simulink model "suijibijin"  (Simulink 7.1)
settings: Solver=ode45  StartTime=0.0  StopTime=200  FixedStep=0.001  RelTol=1e-3  AbsTol=1e-3
libraries: simulink x9
settings Model: Creator=ThinkPad  LastModifiedBy=casi  ExtModeTrigMode=oneshot  ExtModeArmWhenConnect=off
settings DataIOCC: LimitDataPoints=off  SignalLoggingName=sigsOut
settings OptimizationCC: BooleanDataType=off
settings DebuggingCC: SaveWithParameterizedLinksMsg=none  SignalResolutionControl=TryResolveAllWithWarning  SolverPrmCheckMsg=none  MultiTaskDSMMsg=warning  MultiTaskCondExecSysMsg=none  StrictBusMsg=None
settings HardwareCC: TargetUnknown=on
settings RTWCC: IncludeERTFirstTime=on
settings GRTTargetCC: TargetFcnLib=ansi_tfl_tmw.mat

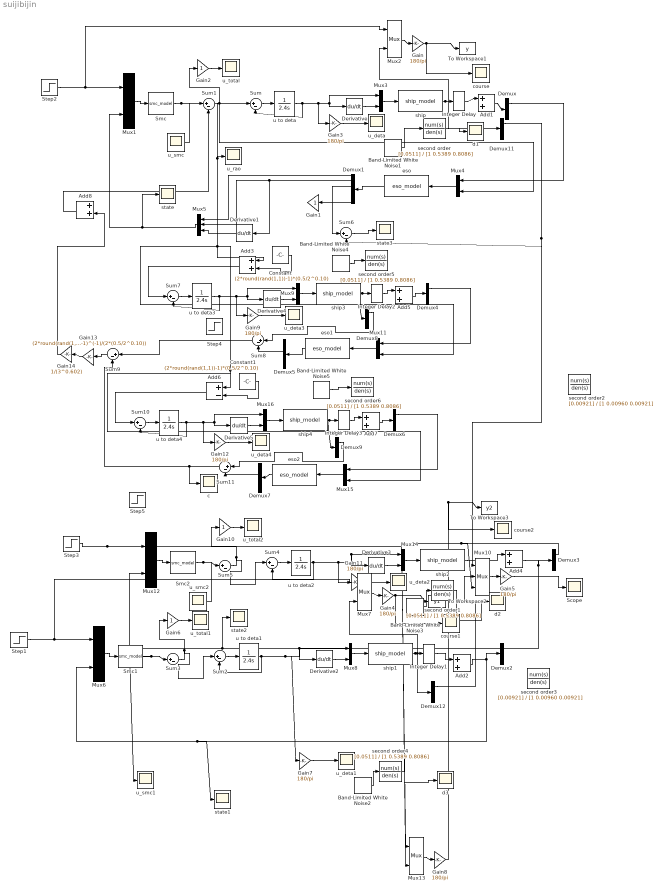
== system suijibijin ==
  Add{1..2,4..5,7} (5 alike) : Sum  OutDataType=sfix(16)  OutScaling=2^-10
  Add3 : Sum  Orientation=left  OutDataType=sfix(16)  OutScaling=2^-10
  Add6 : Sum  Orientation=left  Inputs=+-  OutDataType=sfix(16)  OutScaling=2^-10
  Add8 : Sum  Orientation=left  OutDataType=sfix(16)  OutScaling=2^-10
  Band-Limited White Noise{1..5} (5 alike) : simulink/Sources/Band-Limited White Noise  SystemSampleTime=-1  Cov=[0.01]  Ts=0.1  seed=[23341]
  Constant : Constant  Value=(2*round(rand(1,1))-1)*(0.5/2^0.10)  OutDataType=sfix(16)  OutScaling=2^0
  Constant1 : Constant  Value=(2*round(rand(1,1))-1)*(0.5/2^0.10)  OutDataType=sfix(16)  OutScaling=2^0
  Demux{,2..4,6,8..9,11..12} (9 alike) : Demux  Outputs=3
  Demux1 : Demux  Orientation=left  Outputs=6
  Demux5 : Demux  Orientation=left  Outputs=6
  Demux7 : Demux  Orientation=left  Outputs=6
  Derivative{,2..5} (5 alike) : Derivative
  Derivative1 : Derivative  Orientation=left
  Gain{,3..5,7..9,11..12} (9 alike) : Gain  Gain=180/pi  ParameterDataType=sfix(16)  ParameterScaling=2^0  OutDataType=sfix(16)  OutScaling=2^0
  Gain1 : Gain  Orientation=left  ParameterDataType=sfix(16)  ParameterScaling=2^0  OutDataType=sfix(16)  OutScaling=2^0
  Gain10 : Gain  ParameterDataType=sfix(16)  ParameterScaling=2^0  OutDataType=sfix(16)  OutScaling=2^0
  Gain13 : Gain  Orientation=left  Gain=(2*round(rand(1,1))-1)^(-1)/(2*(0.5/2^0.10))  ParameterDataType=sfix(16)  ParameterScaling=2^0  OutDataType=sfix(16)  OutScaling=2^0
  Gain14 : Gain  Orientation=left  Gain=1/(3^0.602)  ParameterDataType=sfix(16)  ParameterScaling=2^0  OutDataType=sfix(16)  OutScaling=2^0
  Gain2 : Gain  ParameterDataType=sfix(16)  ParameterScaling=2^0  OutDataType=sfix(16)  OutScaling=2^0
  Gain6 : Gain  ParameterDataType=sfix(16)  ParameterScaling=2^0  OutDataType=sfix(16)  OutScaling=2^0
  Integer Delay{,1..3} (4 alike) : simulink/Discrete/Integer Delay  vinit=0.0  samptime=-1  NumDelays=200
  Mux{1..3,6..9,12..14,16} (11 alike) : Mux  Inputs=2
  Mux10 : Mux  Inputs=3
  Mux11 : Mux  Orientation=left  Inputs=2
  Mux15 : Mux  Orientation=left  Inputs=2
  Mux4 : Mux  Orientation=left  Inputs=2
  Mux5 : Mux  Orientation=left  Inputs=3
  Scope : Scope
      settings: YMin=29.985  YMax=30.0125  SaveName=coursebijiao  DataFormat=Array
  Smc : S-Function  FunctionName=smc_model  EnableBusSupport=off
  Smc1 : S-Function  FunctionName=smc_model  EnableBusSupport=off
  Smc2 : S-Function  FunctionName=smc_model  EnableBusSupport=off
  Step1 : Step  Time=0  After=30*pi/180  SampleTime=0  ZeroCross=off
  Step2 : Step  Time=0  After=30*pi/180  SampleTime=0  ZeroCross=off
  Step3 : Step  Time=0  After=30*pi/180  SampleTime=0  ZeroCross=off
  Step4 : Step  Time=0  After=10*pi/180  SampleTime=0  ZeroCross=off
  Step5 : Step  Time=0  After=10*pi/180  SampleTime=0  ZeroCross=off
  Sum{,1..7,10} (9 alike) : Sum  Inputs=|+-  OutDataType=sfix(16)  OutScaling=2^0
  Sum11 : Sum  Orientation=left  Inputs=|+-  OutDataType=sfix(16)  OutScaling=2^0
  Sum8 : Sum  Orientation=left  Inputs=|+-  OutDataType=sfix(16)  OutScaling=2^0
  Sum9 : Sum  Orientation=left  Inputs=|+-  OutDataType=sfix(16)  OutScaling=2^0
  To Workspace1 : ToWorkspace  VariableName=y  SampleTime=-1  SaveFormat=Array
  To Workspace2 : ToWorkspace  VariableName=y1  SampleTime=-1  SaveFormat=Array
  To Workspace3 : ToWorkspace  VariableName=y2  SampleTime=-1  SaveFormat=Array
  c : Scope
      settings: YMin=-0.005  YMax=0.105  SaveName=course3  SampleInput=on
  course : Scope
      settings: YMin=-0.005  YMax=0.105  SaveName=course  SampleInput=on
  course1 : Scope
      settings: YMin=-0.005  YMax=0.105  SaveName=course1  SampleInput=on
  course2 : Scope
      settings: YMin=-0.005  YMax=0.105  SaveName=course2  SampleInput=on
  d1 : Scope
      settings: SaveName=u_total1  SampleInput=on
  d2 : Scope
      settings: SaveName=u_total4  SampleInput=on
  d3 : Scope
      settings: SaveName=u_total2  SampleInput=on
  eso : S-Function  Orientation=left  FunctionName=eso_model  EnableBusSupport=off
  eso1 : S-Function  Orientation=left  FunctionName=eso_model  EnableBusSupport=off
  eso2 : S-Function  Orientation=left  FunctionName=eso_model  EnableBusSupport=off
  second order{,1,4..6} (5 alike) : TransferFcn  Numerator=[0.0511]  Denominator=[1 0.5389 0.8086]
  second order2 : TransferFcn  Numerator=[0.00921]  Denominator=[1 0.00960 0.00921]
  second order3 : TransferFcn  Numerator=[0.00921]  Denominator=[1 0.00960 0.00921]
  ship{,1..4} (5 alike) : S-Function  FunctionName=ship_model  EnableBusSupport=off
  state{,1..3} (4 alike) : Scope
      state settings: SaveName=u_rao1  SampleInput=on
      state1 settings: SaveName=u_rao2  SampleInput=on
      state2 settings: SaveName=u_rao3  SampleInput=on
      state3 settings: SaveName=u_rao4  SampleInput=on
  u to deta{,1..4} (5 alike) : TransferFcn  Denominator=[2.4 0]
  u_deta{,1..4} (5 alike) : Scope
      u_deta settings: TimeRange=100  YMin=2.275e+014  YMax=2.365e+014  SaveName=u_deta  SampleInput=on
      u_deta1 settings: TimeRange=100  YMin=2.275e+014  YMax=2.365e+014  SaveName=u_deta1  SampleInput=on
      u_deta2 settings: TimeRange=100  YMin=2.275e+014  YMax=2.365e+014  SaveName=u_deta2  SampleInput=on
      u_deta3 settings: TimeRange=100  YMin=2.275e+014  YMax=2.365e+014  SaveName=u_deta3  SampleInput=on
      u_deta4 settings: TimeRange=100  YMin=2.275e+014  YMax=2.365e+014  SaveName=u_deta4  SampleInput=on
  u_rao : Scope
      settings: SaveName=u_rao  SampleInput=on
  u_smc : Scope
      settings: SaveName=u_smc  SampleInput=on
  u_smc1 : Scope
      settings: SaveName=u_smc1  SampleInput=on
  u_smc2 : Scope
      settings: SaveName=u_smc2  SampleInput=on
  u_total : Scope
      settings: SaveName=u_total  SampleInput=on
  u_total1 : Scope
      settings: SaveName=u_total3  SampleInput=on
  u_total2 : Scope
      settings: SaveName=u_total5  SampleInput=on
  wires:
  Mux4/1 -> eso/1
  eso/1 -> Demux1/1
  Mux2/1 -> Gain/1
  Smc/1 -> Sum1/1, u_smc/1
  Mux1/1 -> Smc/1
  Step2/1 -> Mux1/1, Mux2/1
  Derivative/1 -> Mux3/2
  Mux3/1 -> ship/1
  Add1/1 -> Demux/1
  ship/1 -> Mux2/2, Integer Delay/1, Demux11/1
  Gain2/1 -> u_total/1
  Gain/1 -> To Workspace1/1, course/1
  Demux/1 -> Mux4/1
  Sum1/1 -> Gain2/1, Mux4/2, Sum/1, Add3/1, Mux11/2, Add6/1, Mux15/2, u_rao/1
  Band-Limited White Noise1/1 -> second order/1
  Gain3/1 -> u_deta/1
  Sum/1 -> u to deta/1
  second order/1 -> d1/1
  Demux1/6 -> Gain1/1
  Mux7/1 -> Gain4/1
  Smc1/1 -> Sum3/1, u_smc1/1
  Mux6/1 -> Smc1/1
  Step1/1 -> Mux6/1, Mux7/1
  Derivative2/1 -> Mux8/2
  Mux8/1 -> ship1/1
  Add2/1 -> Demux2/1, Mux6/2, state1/1
  Gain6/1 -> u_total1/1
  Gain4/1 -> To Workspace2/1, course1/1
  Sum3/1 -> Gain6/1, Sum2/1
  Band-Limited White Noise2/1 -> second order4/1
  Gain7/1 -> u_deta1/1
  Sum2/1 -> u to deta1/1
  u to deta1/1 -> Sum2/2, Mux8/1, Derivative2/1, Gain7/1
  second order4/1 -> d3/1
  Mux10/1 -> Gain5/1
  ship1/1 -> Integer Delay1/1, Mux7/2, Demux12/1
  Integer Delay1/1 -> Add2/1
  Integer Delay/1 -> Add1/1
  Gain5/1 -> Scope/1
  Mux13/1 -> Gain8/1
  Smc2/1 -> Sum5/1, u_smc2/1
  Mux12/1 -> Smc2/1
  Step3/1 -> Mux12/1, Mux13/1
  Derivative3/1 -> Mux14/2
  Mux14/1 -> ship2/1
  Add4/1 -> Demux3/1, Mux12/2, state2/1
  Gain10/1 -> u_total2/1
  Gain8/1 -> To Workspace3/1, course2/1
  Sum5/1 -> Gain10/1, Sum4/1
  Band-Limited White Noise3/1 -> second order1/1
  Gain11/1 -> u_deta2/1
  Sum4/1 -> u to deta2/1
  u to deta2/1 -> Sum4/2, Mux14/1, Derivative3/1, Gain11/1
  second order1/1 -> d2/1
  Demux3/1 -> Mux13/2, Mux10/3
  ship2/1 -> Add4/1
  Constant/1 -> Add3/2
  Mux5/1 -> Mux1/2, state/1
  u to deta/1 -> Mux3/1, Derivative/1, Gain3/1, Sum/2
  Derivative4/1 -> Mux9/2
  Mux9/1 -> ship3/1
  ship3/1 -> Integer Delay2/1, Demux8/1
  Gain9/1 -> u_deta3/1
  Sum7/1 -> u to deta3/1
  u to deta3/1 -> Mux9/1, Derivative4/1, Gain9/1, Sum7/2
  Add3/1 -> Sum7/1
  Demux4/1 -> Mux11/1
  Add5/1 -> Demux4/1
  Mux11/1 -> eso1/1
  eso1/1 -> Demux5/1
  Constant1/1 -> Add6/2
  Derivative5/1 -> Mux16/2
  Mux16/1 -> ship4/1
  Gain12/1 -> u_deta4/1
  Sum10/1 -> u to deta4/1
  u to deta4/1 -> Mux16/1, Derivative5/1, Gain12/1, Sum10/2
  Add6/1 -> Sum10/1
  Demux6/1 -> Mux15/1
  Add7/1 -> Demux6/1
  Mux15/1 -> eso2/1
  eso2/1 -> Demux7/1
  Sum8/1 -> Sum9/1
  Sum11/1 -> Sum9/2, c/1
  Sum9/1 -> Gain13/1
  Gain13/1 -> Gain14/1
  Integer Delay3/1 -> Add7/1
  ship4/1 -> Integer Delay3/1, Demux9/1
  Integer Delay2/1 -> Add5/1
  Add8/1 -> Sum1/2
  Gain14/1 -> Add8/2
  Demux11/1 -> Mux10/1, Sum6/2
  Demux12/1 -> Mux10/2
  Sum6/1 -> state3/1
  Demux1/1 -> Mux5/1
  Demux1/2 -> Mux5/2, Derivative1/1
  Derivative1/1 -> Mux5/3
  Demux1/3 -> Sum6/1
  Demux7/3 -> Sum11/2
  Demux9/1 -> Sum11/1
  Demux5/3 -> Sum8/2
  Demux8/1 -> Sum8/1
  Band-Limited White Noise5/1 -> second order6/1
  Band-Limited White Noise4/1 -> second order5/1
